simulink model "MRFT_CONTROL"  (R2019b)
settings: Solver=FixedStepAuto  StartTime=0.0  StopTime=t_final  FixedStep=time_step  RelTol=1e-3
undefined symbols (not defined in the file or in its folder): beta_mrft, bias_relay, h_mrft, w0
libraries: cstblocks x1, simulink x1
settings Model: SimulationMode=accelerator  Creator=mchehadeh  LastModifiedBy=aaa_b
settings SolverCC: ZeroCrossAlgorithm=Adaptive
settings DataIOCC: LimitDataPoints=on  SaveFormat=Array  ReturnWorkspaceOutputs=off
settings OptimizationCC: BlockReduction=off  BooleanDataType=off  ExpressionDepthLimit=2147483647  LifeSpan=inf
settings DebuggingCC: SaveWithParameterizedLinksMsg=none  UnderspecifiedInitializationDetection=Classic  MergeDetectMultiDrivingBlocksExec=none  SignalResolutionControl=TryResolveAllWithWarning  IgnoredZcDiagnostic=none  MultiTaskDSMMsg=warning  MultiTaskCondExecSysMsg=none  FcnCallInpInsideContextMsg=warning  StateNameClashWarn=warning  SFUnexpectedBacktrackingDiag=warning  SFNoUnconditionalDefaultTransitionDiag=warning  SFExecutionAtInitializationDiag=none  ArithmeticOperatorsInVariantConditions=warning
settings HardwareCC: ProdBitPerPointer=32  ProdBitPerSizeT=32  ProdBitPerPtrDiffT=32  ProdLargestAtomicFloat=None  ProdIntDivRoundTo=Undefined  ProdEndianess=Unspecified  ProdWordSize=32  ProdHWDeviceType=32-bit Generic  TargetUnknown=on
settings ModelReferenceCC: PropagateSignalLabelsOutOfModel=off
settings SFSimCC: SimUseLocalCustomCode=off  CustomCodeUndefinedFunction=UseInterfaceOnly
settings RTWCC: RTWUseLocalCustomCode=off
settings CodeAppCC: StateflowObjectComments=on
settings GRTTargetCC: TargetLangStandard=C89/C90 (ANSI)  GeneratePreprocessorConditionals=Disable all
settings ConfigComp: CovMetricSettings=dw  CovHtmlReporting=on  CovSaveCumulativeToWorkspaceVar=on  CovSaveSingleToWorkspaceVar=on  CovExternalEMLEnable=off

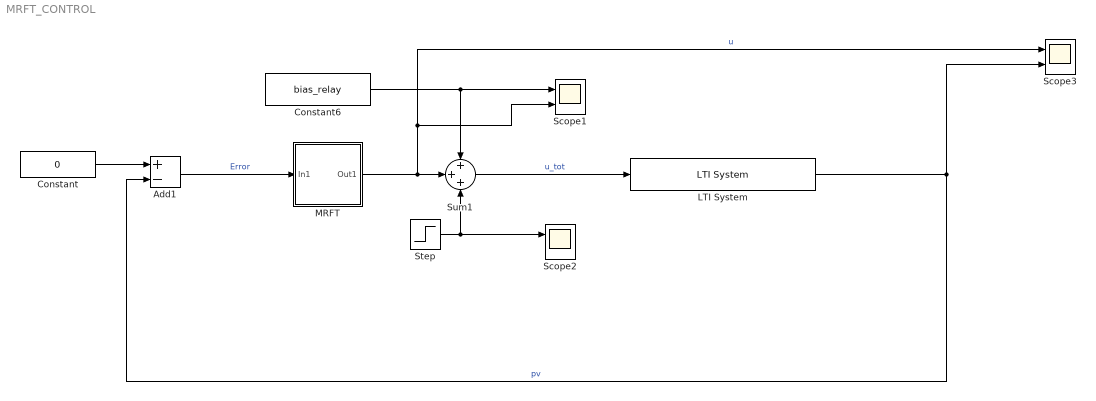
== system MRFT_CONTROL ==
  Add1 : Sum  Inputs=+-
  Constant : Constant  Value=0
  Constant6 : Constant  Value=bias_relay
  LTI System : cstblocks/LTI System  sys=open_loop_sys  IC=[]
  MRFT : Subsystem
  Scope1 : Scope  NumInputPorts=2
  Scope2 : Scope  NumInputPorts=2
  Scope3 : Scope  NumInputPorts=2
  Step : Step  Time=0.0000001  Before=0.000000001  After=0  SampleTime=0
  Sum1 : Sum  Inputs=+++
  wires:
  LTI System/1 -> Add1/2, Scope3/2  "pv"
  Constant/1 -> Add1/1
  Add1/1 -> MRFT/1(In1)  "Error"
  Sum1/1 -> LTI System/1  "u_tot"
  MRFT/1(Out1) -> Sum1/2, Scope1/2, Scope3/1  "u"
  Constant6/1 -> Sum1/1, Scope1/1
  Step/1 -> Scope2/1, Sum1/3

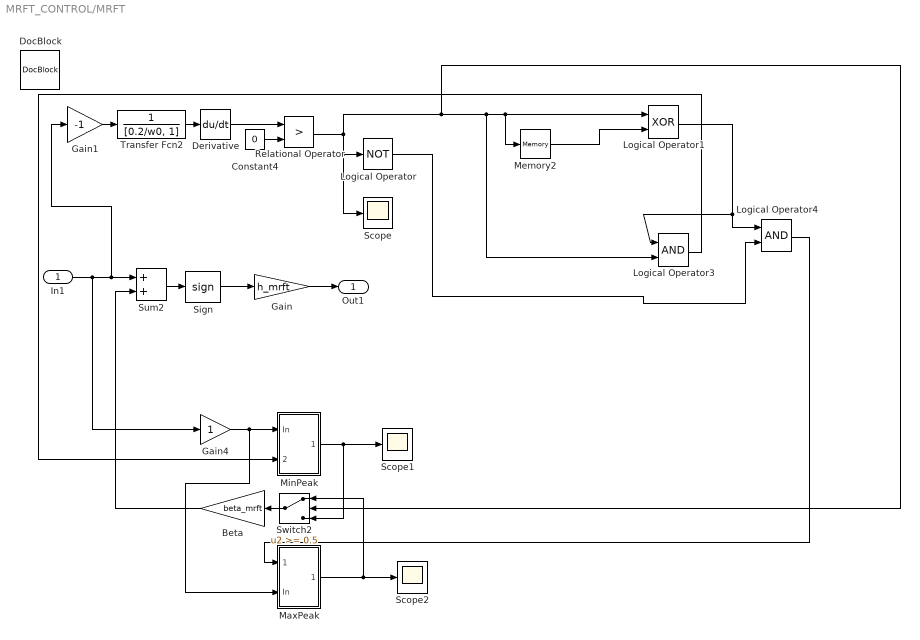
== system MRFT_CONTROL/MRFT ==
  In1 : Inport
  Beta : Gain  Gain=beta_mrft  SaturateOnIntegerOverflow=on  OutDataTypeStr=Inherit: Same as input  ParamDataTypeStr=Inherit: Same as input
  Constant4 : Constant  Value=0
  Derivative : Derivative  CoefficientInTFapproximation=0
  DocBlock : simulink/Model-Wide Utilities/DocBlock  DocumentType=Text
  Gain : Gain  Gain=h_mrft  SaturateOnIntegerOverflow=on  OutDataTypeStr=Inherit: Same as input  ParamDataTypeStr=Inherit: Same as input
  Gain1 : Gain  Gain=-1  SaturateOnIntegerOverflow=on  OutDataTypeStr=Inherit: Same as input  ParamDataTypeStr=Inherit: Same as input
  Gain4 : Gain  SaturateOnIntegerOverflow=on  OutDataTypeStr=Inherit: Same as input  ParamDataTypeStr=Inherit: Same as input
  Logical Operator : Logic  Operator=NOT  Inputs=1
  Logical Operator1 : Logic  Operator=XOR
  Logical Operator3 : Logic
  Logical Operator4 : Logic
  MaxPeak : Subsystem
  Memory2 : Memory
  MinPeak : Subsystem
  Relational Operator : RelationalOperator  Operator=>  RndMeth=Nearest  InputSameDT=on
  Scope : Scope
  Scope1 : Scope
  Scope2 : Scope
  Sign : Signum
  Sum2 : Sum  SaturateOnIntegerOverflow=on  InputSameDT=on  OutDataTypeStr=Inherit: Same as first input
  Switch2 : Switch  Threshold=0.5  SaturateOnIntegerOverflow=on  InputSameDT=on
  Transfer Fcn2 : TransferFcn  Denominator=[0.2/w0, 1]
  Out1 : Outport  VectorParamsAs1DForOutWhenUnconnected=off
  wires:
  Switch2/1 -> Beta/1
  Logical Operator1/1 -> Logical Operator4/1, Logical Operator3/1
  Logical Operator4/1 -> MaxPeak/1(Cntrl)
  Constant4/1 -> Relational Operator/2
  Relational Operator/1 -> Scope/1, Logical Operator/1, Logical Operator1/1, Memory2/1, Logical Operator3/2, Switch2/2
  Logical Operator3/1 -> MinPeak/2(Cntrl)
  Logical Operator/1 -> Logical Operator4/2
  Sign/1 -> Gain/1
  Gain4/1 -> MinPeak/1(In), MaxPeak/2(In)
  Sum2/1 -> Sign/1
  Beta/1 -> Sum2/2
  MaxPeak/1(Out) -> Scope2/1, Switch2/1
  MinPeak/1(Out) -> Scope1/1, Switch2/3
  Derivative/1 -> Relational Operator/1
  Gain/1 -> Out1/1
  In1/1 -> Gain4/1, Gain1/1, Sum2/1
  Memory2/1 -> Logical Operator1/2
  Gain1/1 -> Transfer Fcn2/1
  Transfer Fcn2/1 -> Derivative/1

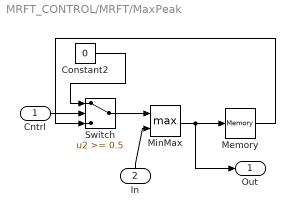
== system MRFT_CONTROL/MRFT/MaxPeak ==
  Cntrl : Inport
  In : Inport  Port=2
  Constant2 : Constant  Value=0
  Memory : Memory
  MinMax : MinMax  Function=max  Inputs=2  SaturateOnIntegerOverflow=on  InputSameDT=on
  Switch : Switch  Threshold=0.5  SaturateOnIntegerOverflow=on  InputSameDT=on
  Out : Outport  VectorParamsAs1DForOutWhenUnconnected=off
  wires:
  MinMax/1 -> Memory/1, Out/1
  Switch/1 -> MinMax/1
  Constant2/1 -> Switch/1
  Memory/1 -> Switch/3
  In/1 -> MinMax/2
  Cntrl/1 -> Switch/2

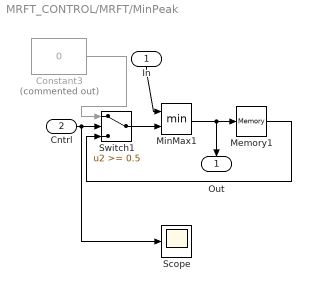
== system MRFT_CONTROL/MRFT/MinPeak ==
  In : Inport
  Cntrl : Inport  Port=2
  Constant3 : Constant  Commented=on  Value=0
  Memory1 : Memory
  MinMax1 : MinMax  Inputs=2  SaturateOnIntegerOverflow=on  InputSameDT=on
  Scope : Scope
  Switch1 : Switch  Threshold=0.5  SaturateOnIntegerOverflow=on  InputSameDT=on
  Out : Outport  VectorParamsAs1DForOutWhenUnconnected=off
  wires:
  MinMax1/1 -> Memory1/1, Out/1
  Switch1/1 -> MinMax1/2
  Memory1/1 -> Switch1/3
  Constant3/1 -> Switch1/1
  In/1 -> MinMax1/1
  Cntrl/1 -> Switch1/2, Scope/1
